simulink model "top_model"  (R2017a)
settings: Solver=VariableStepAuto  StartTime=0.0  StopTime=150  RelTol=1e-3  EnableMultiTasking=on
undefined symbols (not defined in the file): cb, cf, db, df, g, h, I0, Ib, If, kb, kf, m, n, rb, rf
libraries: simulink x4
settings Model: Creator=The MathWorks, Inc.  LastModifiedBy=Till
settings DataIOCC: LimitDataPoints=on
settings OptimizationCC: LifeSpan=inf
settings DebuggingCC: AllowSymbolicDim=off  SFUnexpectedBacktrackingDiag=warning  SFNoUnconditionalDefaultTransitionDiag=warning  SFExecutionAtInitializationDiag=none
settings ModelReferenceCC: PropagateSignalLabelsOutOfModel=off
settings GRTTargetCC: TargetLangStandard=C89/C90 (ANSI)
settings ConfigComp: CovMetricSettings=dw  CovHtmlReporting=on  CovSaveCumulativeToWorkspaceVar=on  CovSaveSingleToWorkspaceVar=on  CovExternalEMLEnable=off

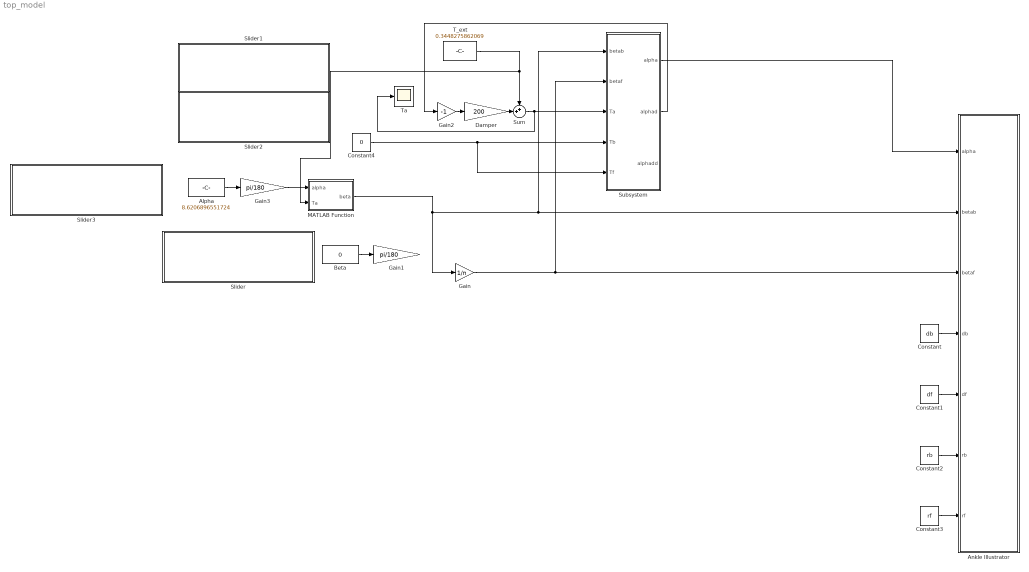
== system top_model ==
  Alpha : Constant  Value=8.6206896551724
  Ankle Illustrator : MATLAB Function  TreatAsAtomicUnit=on
  Beta : Constant  Value=0
  Constant : Constant  Value=db
  Constant1 : Constant  Value=df
  Constant2 : Constant  Value=rb
  Constant3 : Constant  Value=rf
  Constant4 : Constant  Value=0
  Damper : Gain  Gain=200
  Gain : Gain  Gain=1/n
  Gain1 : Gain  Gain=pi/180
  Gain2 : Gain  Gain=-1
  Gain3 : Gain  Gain=pi/180
  MATLAB Function : MATLAB Function  TreatAsAtomicUnit=on
  Slider : Subsystem  DialogController=hmiCreateDDGDialog  IsWebBlock=on  mask(MWDashboardBlock){webBlockId=7d47b49e-c981-4ea1-8dee-4c091c406145, webBlockType=slider, ShowInLibBrowser=on, ShowInitialText=on, HMISrcModelName=top_model}
      mask prompts: webBlockId "WebBlock Id"; webBlockType "WebBlock Type"; HMISrcModelName "Source Model"
      mask help: SimulinkHMI:dialogs:SliderDialogDesc
      mask Help: helpview([docroot '/mapfiles/simulink.map'], 'hmi_slider')
      mask Display:
      | if strcmp(get_param(bdroot(gcb),'BlockDiagramType'), 'library')
      |     image([(matlabroot) '/toolbox/simulink/hmi/icons/Slider.png']);
      | end
  Slider1 : Subsystem  DialogController=hmiCreateDDGDialog  IsWebBlock=on  mask(MWDashboardBlock){webBlockId=8b13a410-a01c-40ec-aacb-68b803189e65, webBlockType=slider, ShowInLibBrowser=on, ShowInitialText=on, HMISrcModelName=top_model}
      mask prompts: webBlockId "WebBlock Id"; webBlockType "WebBlock Type"; HMISrcModelName "Source Model"
      mask help: SimulinkHMI:dialogs:SliderDialogDesc
      mask Help: helpview([docroot '/mapfiles/simulink.map'], 'hmi_slider')
      mask Display:
      | if strcmp(get_param(bdroot(gcb),'BlockDiagramType'), 'library')
      |     image([(matlabroot) '/toolbox/simulink/hmi/icons/Slider.png']);
      | end
  Slider2 : Subsystem  DialogController=hmiCreateDDGDialog  IsWebBlock=on  mask(MWDashboardBlock){webBlockId=728ae993-fdbe-4a5b-b338-448b75d674bd, webBlockType=slider, ShowInLibBrowser=on, ShowInitialText=on, HMISrcModelName=top_model}
      mask prompts: webBlockId "WebBlock Id"; webBlockType "WebBlock Type"; HMISrcModelName "Source Model"
      mask help: SimulinkHMI:dialogs:SliderDialogDesc
      mask Help: helpview([docroot '/mapfiles/simulink.map'], 'hmi_slider')
      mask Display:
      | if strcmp(get_param(bdroot(gcb),'BlockDiagramType'), 'library')
      |     image([(matlabroot) '/toolbox/simulink/hmi/icons/Slider.png']);
      | end
  Slider3 : Subsystem  DialogController=hmiCreateDDGDialog  IsWebBlock=on  mask(MWDashboardBlock){webBlockId=5321fe2c-e6bd-4293-bd6a-348a93fc8914, webBlockType=slider, ShowInLibBrowser=on, ShowInitialText=on, HMISrcModelName=top_model}
      mask prompts: webBlockId "WebBlock Id"; webBlockType "WebBlock Type"; HMISrcModelName "Source Model"
      mask help: SimulinkHMI:dialogs:SliderDialogDesc
      mask Help: helpview([docroot '/mapfiles/simulink.map'], 'hmi_slider')
      mask Display:
      | if strcmp(get_param(bdroot(gcb),'BlockDiagramType'), 'library')
      |     image([(matlabroot) '/toolbox/simulink/hmi/icons/Slider.png']);
      | end
  Subsystem : Subsystem
  Sum : Sum  Inputs=++|
  "T_ext " : Constant  Value=0.3448275862069
  Ta : Scope
  wires:
  Subsystem/1("alpha ") -> Ankle Illustrator/1(alpha)
  Constant/1 -> Ankle Illustrator/4(db)
  Constant1/1 -> Ankle Illustrator/5(df)
  Constant2/1 -> Ankle Illustrator/6(rb)
  Constant3/1 -> Ankle Illustrator/7(rf)
  Gain/1 -> Subsystem/2(betaf), Ankle Illustrator/3(betaf)
  Constant4/1 -> Subsystem/5(Tf), Subsystem/4(Tb)
  Subsystem/2(alphad) -> Gain2/1
  "T_ext "/1 -> MATLAB Function/2(Ta), Sum/1
  Damper/1 -> Sum/2
  Sum/1 -> Ta/1, Subsystem/3(Ta)
  MATLAB Function/1(beta) -> Gain/1, Subsystem/1(betab), Ankle Illustrator/2(betab)
  Gain2/1 -> Damper/1
  Alpha/1 -> Gain3/1
  Gain3/1 -> MATLAB Function/1(alpha)
  Beta/1 -> Gain1/1

== system top_model/Slider ==

== system top_model/Slider1 ==

== system top_model/Slider2 ==

== system top_model/Slider3 ==

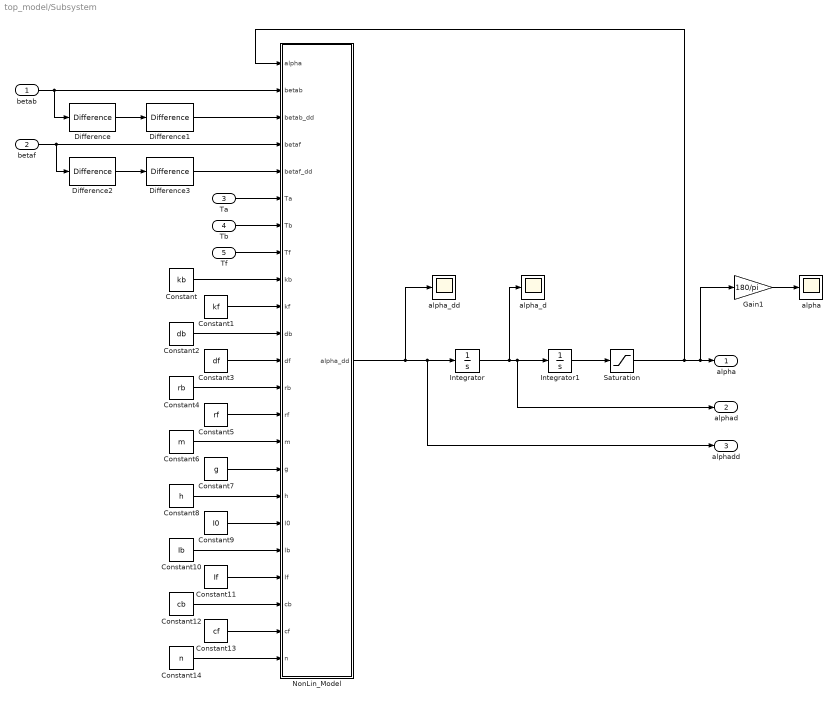
== system top_model/Subsystem ==
  betab : Inport
  betaf : Inport  Port=2
  Ta : Inport  Port=3
  Tb : Inport  Port=4
  Tf : Inport  Port=5
  Constant : Constant  Value=kb
  Constant1 : Constant  Value=kf
  Constant10 : Constant  Value=Ib
  Constant11 : Constant  Value=If
  Constant12 : Constant  Value=cb
  Constant13 : Constant  Value=cf
  Constant14 : Constant  Value=n
  Constant2 : Constant  Value=db
  Constant3 : Constant  Value=df
  Constant4 : Constant  Value=rb
  Constant5 : Constant  Value=rf
  Constant6 : Constant  Value=m
  Constant7 : Constant  Value=g
  Constant8 : Constant  Value=h
  Constant9 : Constant  Value=I0
  Difference{,1..3} (4 alike) : simulink/Discrete/Difference  ICPrevInput=0  OutMin=[]  OutMax=[]  OutDataType=fixdt(1, 16)  OutScaling=2^-10  DoSatur=off
  Gain1 : Gain  Gain=180/pi
  Integrator : Integrator
  Integrator1 : Integrator
  NonLin_Model : MATLAB Function  TreatAsAtomicUnit=on
  Saturation : Saturate  UpperLimit=pi/180*45  LowerLimit=-pi/180*45
  alpha : Scope
  alpha_d : Scope
  alpha_dd : Scope
  "alpha " : Outport
  alphad : Outport  Port=2
  alphadd : Outport  Port=3
  wires:
  Integrator/1 -> alpha_d/1, alphad/1, Integrator1/1
  Integrator1/1 -> Saturation/1
  betab/1 -> Difference/1, NonLin_Model/2(betab)
  Tb/1 -> NonLin_Model/7(Tb)
  betaf/1 -> Difference2/1, NonLin_Model/4(betaf)
  Ta/1 -> NonLin_Model/6(Ta)
  Constant1/1 -> NonLin_Model/10(kf)
  Constant/1 -> NonLin_Model/9(kb)
  Constant2/1 -> NonLin_Model/11(db)
  Constant3/1 -> NonLin_Model/12(df)
  Constant4/1 -> NonLin_Model/13(rb)
  Constant5/1 -> NonLin_Model/14(rf)
  Constant6/1 -> NonLin_Model/15(m)
  Constant7/1 -> NonLin_Model/16(g)
  Constant8/1 -> NonLin_Model/17(h)
  Tf/1 -> NonLin_Model/8(Tf)
  Constant9/1 -> NonLin_Model/18(I0)
  Constant10/1 -> NonLin_Model/19(Ib)
  Constant11/1 -> NonLin_Model/20(If)
  Difference/1 -> Difference1/1
  Difference2/1 -> Difference3/1
  Constant12/1 -> NonLin_Model/21(cb)
  Constant13/1 -> NonLin_Model/22(cf)
  Constant14/1 -> NonLin_Model/23(n)
  Difference1/1 -> NonLin_Model/3(betab_dd)
  Difference3/1 -> NonLin_Model/5(betaf_dd)
  NonLin_Model/1(alpha_dd) -> alpha_dd/1, alphadd/1, Integrator/1
  Gain1/1 -> alpha/1
  Saturation/1 -> NonLin_Model/1(alpha), Gain1/1, "alpha "/1

== matlab function top_model/Subsystem/NonLin_Model ==
  data: alpha input; alpha_dd output; betab input; betab_dd input; betaf input; betaf_dd input; Ta input; Tb input; Tf input; kb input; kf input; db input; df input; rb input; rf input; m input; g input; h input; I0 input; Ib input; If input; cb input; cf input; n input
function alpha_dd = fcn(alpha, betab, betab_dd, betaf, betaf_dd,...
                        Ta, Tb, Tf,...
                        kb,kf,db,df,rb,rf,m,g,h,I0,Ib,If,cb,cf,n)

 lambda=(If*betaf_dd + kf*(cf+ betaf*rf - sin(alpha)*df)*rf - n*Ib*betab_dd -n*kb*(cb+ betab*rb - sin(alpha)*db)*rb + n*Tb -Tf)/(cos(alpha)*(kf*df*rf + n*kb*db*rb));
 
 alpha_dd=1/I0 * (cos(alpha)*m*g*h + kb*(cb + betab*rb - sin(alpha)*db)*cos(alpha)*db + kf*(cf+ betaf*rf - sin(alpha)*df)*cos(alpha)*df ...
            + lambda*(-sin(alpha)*(kf*df*(cf +betaf*rf ) - kb*db*(cb + betab* rb))+2*cos(2*alpha)*(kb*db^2 - kf*df^2)) +Ta);
        
end

== matlab function top_model/Ankle Illustrator ==
  data: alpha input; betab input; betaf input; db input; df input; rb input; rf input
function fcn(alpha,betab,betaf,db,df,rb,rf)


clf
hold on;
rotCenter = [0;0];

s=0.5;
l_lower=0.1*s;
l_upper=0.4*s;

A = rotCenter + [cos(alpha),sin(alpha);-sin(alpha),cos(alpha)]*[-db; 0]; %back end of ankle bar
B = rotCenter + [cos(alpha),sin(alpha);-sin(alpha),cos(alpha)]*[df; 0];  %front end of ankle bar

C = rotCenter + [-db+rb; s];    %center hoist in back
D = rotCenter + [df-rf; s];     %center hoist in front

vb = (C-[rb;0]-A)/norm(C-[rb;0]-A);
vf = (D+[rf;0]-B)/norm(D+[rf;0]-B);

plot([A(1),B(1)],[A(2),B(2)],'b-')
plot([rotCenter(1)-db, rotCenter(1)+df],[rotCenter(2),rotCenter(2)],'k--')

[x,y]=circle(C(1),C(2),rb);
plot(x,y,'b-')
vr=[-rb*1.5;0];
plot([C(1),C(1)+vr(1)],[C(2),C(2)+vr(2)],'k--')
vr=[cos(betab),sin(betab);-sin(betab),cos(betab)]*vr;
plot([C(1),C(1)+vr(1)],[C(2),C(2)+vr(2)],'k-')

[x,y]=circle(D(1),D(2),rf);
plot(x,y,'b-')
vr=[rf*1.5;0];
plot([D(1),D(1)+vr(1)],[D(2),D(2)+vr(2)],'k--')
vr=[cos(betaf),sin(betaf);-sin(betaf),cos(betaf)]*vr;
plot([D(1),D(1)+vr(1)],[D(2),D(2)+vr(2)],'k-')



%Back String + Spring
p1=A;
p2=A+vb*l_lower;
p3=C-[rb;0]-vb*(l_upper-betab*rb);
p4=C-[rb;0];
[x,y]=spring(p2(1),p2(2),p3(1),p3(2),20,s*1.1,0.01);

plot([p1(1),p2(1)],[p1(2),p2(2)],'b-');
plot(x,y,'r-');
plot([p3(1),p4(1)],[p3(2),p4(2)],'b-');

%Front String + Spring
p1=B;
p2=B+vf*l_lower;
p3=D+[rf;0]-vf*(l_upper+betaf*rf);
p4=D+[rf;0];
[x,y]=spring(p2(1),p2(2),p3(1),p3(2),20,s*1.1,0.01);

plot([p1(1),p2(1)],[p1(2),p2(2)],'b-');
plot(x,y,'r-');
plot([p3(1),p4(1)],[p3(2),p4(2)],'b-');


a=s*1.3/2;
axis([-a a -s*0.2 s*1.1])

drawnow
end

== matlab function top_model/MATLAB Function ==
  data: alpha input; beta output; Ta input
function beta = fcn(alpha, Ta)

beta = -(Ta - 1000*sin(2*alpha) + (981*cos(alpha))/250)/(400*cos(alpha));
